simulink model "Ex3_3_x2_StateSpace_sim"  (R2015a)
settings: Solver=ode45  StartTime=0.0  StopTime=0.2  RelTol=1e-3
values from neighbouring files (symbols this model uses):
  A = [-R/L, -K_e/L; K_t/J, -D/J]    [Ex3_3_x2_StateSpace.m]
  b = [1/L, 0]'    [Ex3_3_x2_StateSpace.m]
  c = [0, 1]    [Ex3_3_x2_StateSpace.m]
  d = 0    [Ex3_3_x2_StateSpace.m]
settings Model: CovSFcnEnable=off  Creator=Shin  LastModifiedBy=Shin
settings DebuggingCC: SolverPrmCheckMsg=warning

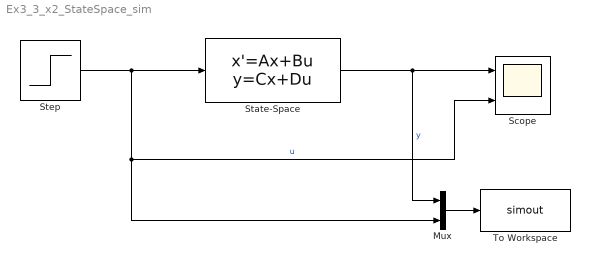
== system Ex3_3_x2_StateSpace_sim ==
  Mux : Mux  Inputs=2
  Scope : Scope  NumInputPorts=2
      settings: YMin=0~0  YMax=0.3~2
  State-Space : StateSpace  A=A  B=b  C=c  D=d  X0=0
  Step : Step  Time=0.01  After=u  SampleTime=0
  To Workspace : ToWorkspace  VariableName=simout  SaveFormat=Timeseries  SampleTime=-1
  wires:
  State-Space/1 -> Mux/1, Scope/1  "y"
  Step/1 -> State-Space/1, Scope/2, Mux/2  "u"
  Mux/1 -> To Workspace/1
